simulink model "Acrobot_test"  (R2022b)
settings: Solver=FixedStepAuto  StartTime=0  StopTime=60  FixedStep=0.001  RelTol=1e-2  AbsTol=1e-3  EnableMultiTasking=on
undefined symbols (not defined in the file): AL1, AL2, Alink1_CM, Alink1_m, Alink1_MI, Alink1_PI, Alink2_CM, Alink2_m, Alink2_MI, Alink2_PI, H, W, X, Y, Z
libraries: nesl_utility x19, sm_lib x12
settings Model: Creator=李东昊  LastModifiedBy=dong
settings SolverCC: AutoScaleAbsTol=off  AlgebraicLoopSolver=TrustRegion  MaxZcPerStep=1
settings DataIOCC: LimitDataPoints=on  MaxDataPoints=10000
settings OptimizationCC: LifeSpan=inf
settings DebuggingCC: UnconnectedInputMsg=warning  UnconnectedOutputMsg=warning  UnconnectedLineMsg=warning  AllowSymbolicDim=off  SFUnexpectedBacktrackingDiag=warning  SFNoUnconditionalDefaultTransitionDiag=warning  SFExecutionAtInitializationDiag=none  SFMachineParentedDataDiag=warning  ArithmeticOperatorsInVariantConditions=warning
settings ModelReferenceCC: EnableRefExpFcnMdlSchedulingChecks=on
settings SFSimCC: SimUseLocalCustomCode=off  CustomCodeUndefinedFunction=UseInterfaceOnly
settings RTWCC: RTWUseLocalCustomCode=off  DLArmComputeVersion=19.05
settings CodeAppCC: StateflowObjectComments=on
settings GRTTargetCC: TargetLangStandard=C89/C90 (ANSI)
settings ConfigComp: CovMetricSettings=dw  CovSaveCumulativeToWorkspaceVar=on  CovSaveSingleToWorkspaceVar=on  CovExternalEMLEnable=off  CovSFcnEnable=off
settings SimscapeCC: SimscapeLogType=all  SimscapeLogSimulationStatistics=on  SimscapeLogDataHistory=10000
settings ExplorerConfigSet: InternalSimMechanicsExplorerSettings="<ExplorerConfiguration><canonicalview>aerospace</canonicalview><AnimationSetting><BasePlaybackSpeed>1.0</BasePlaybackSpeed><PlaybackSpeedFactor>1.0</PlaybackSpeedFactor></AnimationSetting><TilePanel><TileInfo><Tiles Columns=\"1\" Count=\"1\" Rows=\"1\"><Column Weight=\"1\"/><Row Weight=\"1\"/><Tile Height=\"1\" Width=\"1\" X=\"0\" Y=\"0\"/></Tiles></TileInfo><SceneInfo><SceneViewer><BGColor><R>0.60000002384185791</R><G>0.60000002384185791</G><B>0.60000002384185791</B></BGColor><Camera><DoPerspective>off</DoPerspective><Position><X>-0.471212034882517727</X><Y>0.213512906624389098</Y><Z>1.00000005247557366</Z></Position><Center><X>-0.471212034882517727</X><Y>0.213512906624389098</Y><Z>5.24755735531456935e-08</Z></Center><Up><X>0</X><Y>1</Y><Z>0</Z></Up><ViewLimDist>1</ViewLimDist><YLim>1.41406501065933288</YLim><XLim>1.62924881662923138</XLim></Camera></SceneViewer></SceneInfo></TilePanel><MechEditorPanel><Cameras/><GfxPanelCameraMap/><VideoCreator><PlaybackSpeedRatio>1.0</PlaybackSpeedRatio><FrameRate>30</FrameRate><VideoFormat>MPEG-4</VideoFormat><FrameSize>[800 600]</FrameSize></VideoCreator></MechEditorPanel></ExplorerConfiguration>"

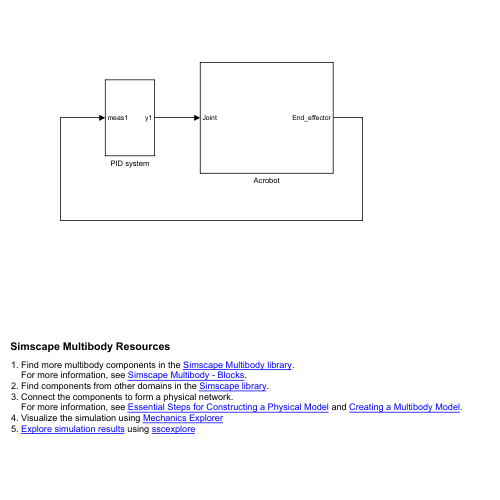
[thumbnail: Simulink's stored preview of the top-level diagram]
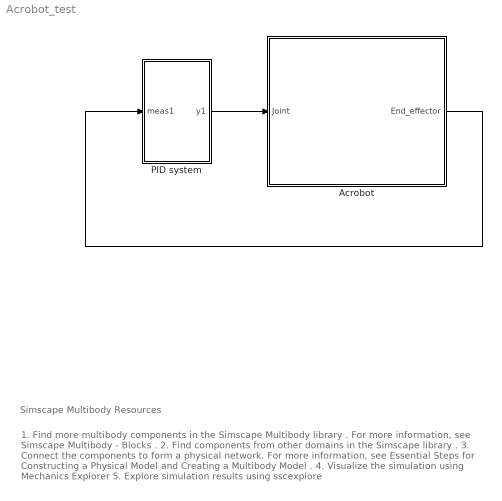
== system Acrobot_test ==
  note: 1. Find more multibody components in the Simscape Multibody library .
      | For more information, see Simscape Multibody - Blocks .
      | 2. Find components from other domains in the Simscape library .
      | 3. Connect the components to form a physical network.
      | For more information, see Essential Steps for Constructing a Physical Model and Creating a Multibody Model .
      | 4. Visualize the simulation using Mechanics Explorer
      | 5. Explore simulation results using sscexplore
  note: Simscape Multibody Resources
  Acrobot : Subsystem
  PID system : Subsystem
  wires:
  Acrobot/1(End_effector) -> PID system/1(meas1)
  PID system/1(y1) -> Acrobot/1(Joint)

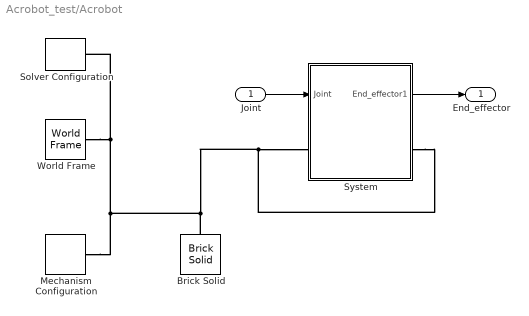
== system Acrobot_test/Acrobot ==
  Joint : Inport
  Brick Solid : sm_lib/Body Elements/Brick Solid  GraphicAmbientColor=[0.15 0.15 0.15 1.0]  BasedOnType=Density  BrickDimensions=[0.1 0.1 0.1]  BrickDimensionUnits=m  CenterOfMass=[0 0 0]  CenterOfMassUnits=m  GraphicDiffuseColor=[0.5 0.5 0.5]  Density=1000  DensityUnits=kg/m^3  DoExposeReferenceFrame=on  GraphicEmissiveColor=[0.0 0.0 0.0 1.0]  ExportEntireGeometry=off  SerializedFrames=<Frames/>  MarkerShape=Sphere  MarkerSize=10  GraphicType=FromGeometry  InertiaType=CalculateFromGeometry  Mass=1  MassUnits=kg  MomentsOfInertia=[1 1 1]  MomentsOfInertiaUnits=kg*m^2  GraphicOpacity=1.0  ProductsOfInertia=[0 0 0]  ProductsOfInertiaUnits=kg*m^2  GraphicShininess=75  GraphicSpecularColor=[0.5 0.5 0.5 1.0]  GraphicVisPropType=SimpleVisualProperties
  Mechanism Configuration : sm_lib/Utilities/Mechanism Configuration  UniformGravity=Constant  GravityVector=[0 -9.81 0]  GravityUnits=m/s^2  LinearizationDelta=0.001  JointModeTransitionNonlinearIterations=2
  Solver Configuration : nesl_utility/Solver Configuration  PhysicalDomain=network_engine_domain  SubClassName=solver  LeftPortType=input  RightPortType=generic  Tones=[]  Harmonics=[]  SimulateNoise=off  Profile=off  UseLocalSampling=off  EnableSwitchedLinearOptims=on  FrequencyDomain=off  UseCCode=off  RelTol=0.001  AbsTol=1e-06  MinStep=1e-09  ToWorkspace=off  RevertToSquareIcSolve=off  NumHomotopyIterations=100  PhasorMode=off  PhasorModeNumHarmonics=1  ConsistencySolver=NEWTON_FTOL  IndexReductionMethod=DerivativeReplacement  DoDC=off  ResidualTolerance=1e-09  ConsistencyTolSource=GLOBAL  ConsistencyAbsTol=0.001  ConsistencyRelTol=0.001  ConsistencyTolFactor=0.001  UseLocalSolver=off  LocalSolverChoice=NE_BACKWARD_EULER_ADVANCER  ResolveIndetEquations=on  FunctionEvalNumThread=1  LocalSolverSampleTime=0.001  DoFixedCost=off  MaxNonlinIter=3  MaxModeIter=2  ComputeImpulses=off  ImpulseIterations=2  LinearAlgebra=Sparse  LinearAlgebraNumThread=0  EquationFormulation=NE_TIME_EF  DelaysMemoryBudget=1024  AutomaticFiltering=on  FilteringTimeConstant=0.001  PartitionStorageMethod=AS_NEEDED  PartitionMemoryBudget=1024  PartitionMethod=FAST
  System : Subsystem
  World Frame : sm_lib/Frames and Transforms/World Frame
  End_effector : Outport
  wires:
  Joint/1 -> System/1(Joint)
  System/1(End_effector1) -> End_effector/1
  connections:
  System/LConn1 -- System/RConn1 -- Brick Solid/RConn1 -- World Frame/RConn1 -- Solver Configuration/RConn1 -- Mechanism Configuration/RConn1

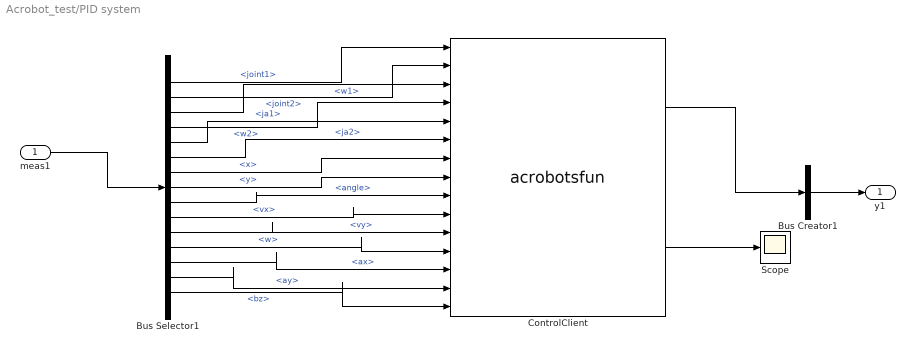
== system Acrobot_test/PID system ==
  meas1 : Inport
  Bus Creator1 : BusCreator  Inputs=1
  Bus Selector1 : BusSelector  OutputSignals=joint1,joint2,w1,w2,ja1,ja2,signal1.x,signal1.y,signal1.angle,signal1.vx,signal1.vy,signal1.w,signal1.ax,signal1.ay,signal1.bz
  ControlClient : S-Function  FunctionName=acrobotsfun  Parameters=hostname,portname,stepsize,inputnum,outputnum  SFunctionDeploymentMode=off  EnableBusSupport=off  mask{hostname=localhost, portname=8099, stepsize=0.001, inputnum=15, outputnum=2}
      mask prompts: hostname "host"; portname "port"; stepsize "step"; inputnum "input num"; outputnum "output num"
      mask DialogControl ParameterGroupVar Prompt: 参数
      mask Display:
      | color('red');
      | image('Simulink_Logo.png');
  Scope : Scope
  y1 : Outport
  wires:
  Bus Creator1/1 -> y1/1
  meas1/1 -> Bus Selector1/1
  ControlClient/1 -> Bus Creator1/1
  Bus Selector1/1 -> ControlClient/1  "<joint1>"
  Bus Selector1/2 -> ControlClient/2  "<joint2>"
  Bus Selector1/3 -> ControlClient/3  "<w1>"
  Bus Selector1/4 -> ControlClient/4  "<w2>"
  Bus Selector1/7 -> ControlClient/7  "<x>"
  Bus Selector1/8 -> ControlClient/8  "<y>"
  Bus Selector1/9 -> ControlClient/9  "<angle>"
  Bus Selector1/10 -> ControlClient/10  "<vx>"
  Bus Selector1/11 -> ControlClient/11  "<vy>"
  Bus Selector1/12 -> ControlClient/12  "<w>"
  Bus Selector1/13 -> ControlClient/13  "<ax>"
  Bus Selector1/14 -> ControlClient/14  "<ay>"
  Bus Selector1/15 -> ControlClient/15  "<bz>"
  Bus Selector1/6 -> ControlClient/6  "<ja2>"
  Bus Selector1/5 -> ControlClient/5  "<ja1>"
  ControlClient/2 -> Scope/1

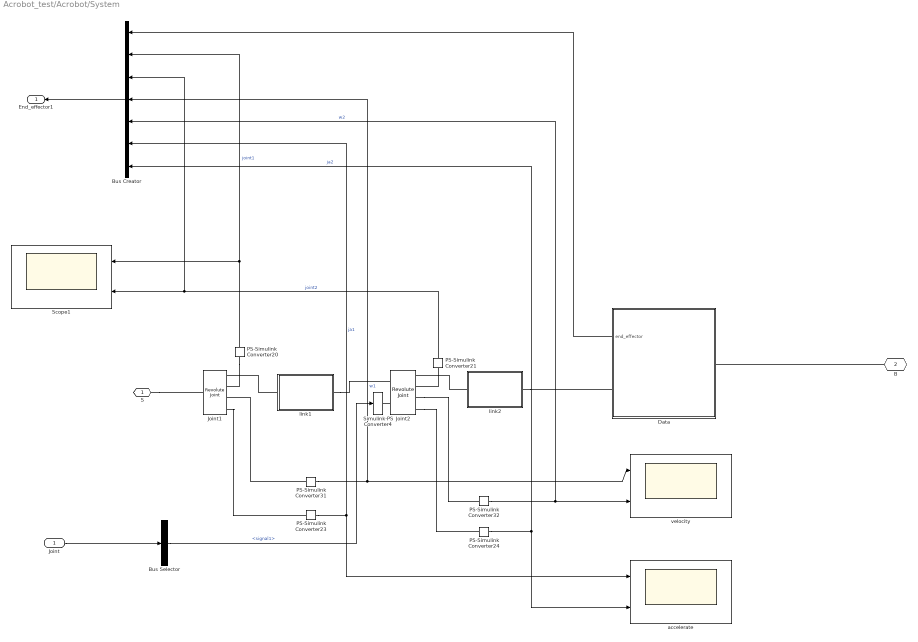
== system Acrobot_test/Acrobot/System ==
  Joint : Inport
  Bus Creator : BusCreator  Inputs=7
  Bus Selector : BusSelector  OutputSignals=signal1
  Data : Subsystem
  Joint1 : sm_lib/Joints/Revolute Joint  JointMode=Normal  SenseConstraintForce=off  SenseConstraintForceX=off  SenseConstraintForceY=off  SenseConstraintForceZ=off  SenseConstraintTorque=off  SenseConstraintTorqueX=off  SenseConstraintTorqueY=off  SenseConstraintTorqueZ=off  SenseTotalForce=off  SenseTotalForceX=off  SenseTotalForceY=off  SenseTotalForceZ=off  SenseTotalTorque=off  SenseTotalTorqueX=off  SenseTotalTorqueY=off  SenseTotalTorqueZ=off  CompositeWrenchDir=BaseOnFollower  CompositeWrenchFrame=BaseFrame  EquilibriumPosition=0  EquilibriumPositionUnits=deg  SpringStiffness=0  SpringStiffnessUnits=N*m/deg  DampingCoefficient=0  DampingCoefficientUnits=N*m/(deg/s)  TorqueActuationMode=NoTorque  MotionActuationMode=ComputedMotion  SensePosition=on  SenseVelocity=on  SenseAcceleration=on  SenseTorqueForce=off  SenseLowerLimitTorqueForce=off  SenseUpperLimitTorqueForce=off  LowerLimitSpecify=off  LowerLimitBound=-90  LowerLimitBoundUnits=deg  LowerLimitStiffness=1e4  LowerLimitStiffnessUnits=N*m/deg  LowerLimitDamping=10  LowerLimitDampingUnits=N*m/(deg/s)  LowerLimitTransitionRegionWidth=0.1  LowerLimitTransitionRegionWidthUnits=deg  UpperLimitSpecify=off  UpperLimitBound=90  UpperLimitBoundUnits=deg  UpperLimitStiffness=1e4  UpperLimitStiffnessUnits=N*m/deg  UpperLimitDamping=10  UpperLimitDampingUnits=N*m/(deg/s)  UpperLimitTransitionRegionWidth=0.1  UpperLimitTransitionRegionWidthUnits=deg  PositionTargetSpecify=off  PositionTargetPriority=High  PositionTargetValue=2.813628238  PositionTargetValueUnits=rad  VelocityTargetSpecify=off  VelocityTargetPriority=Low  VelocityTargetValue=0  VelocityTargetValueUnits=rad/s
  Joint2 : sm_lib/Joints/Revolute Joint  JointMode=Normal  SenseConstraintForce=off  SenseConstraintForceX=off  SenseConstraintForceY=off  SenseConstraintForceZ=off  SenseConstraintTorque=off  SenseConstraintTorqueX=off  SenseConstraintTorqueY=off  SenseConstraintTorqueZ=off  SenseTotalForce=off  SenseTotalForceX=off  SenseTotalForceY=off  SenseTotalForceZ=off  SenseTotalTorque=off  SenseTotalTorqueX=off  SenseTotalTorqueY=off  SenseTotalTorqueZ=off  CompositeWrenchDir=BaseOnFollower  CompositeWrenchFrame=BaseFrame  EquilibriumPosition=0  EquilibriumPositionUnits=deg  SpringStiffness=0  SpringStiffnessUnits=N*m/deg  DampingCoefficient=0  DampingCoefficientUnits=N*m/(deg/s)  TorqueActuationMode=InputTorque  MotionActuationMode=ComputedMotion  SensePosition=on  SenseVelocity=on  SenseAcceleration=on  SenseTorqueForce=off  SenseLowerLimitTorqueForce=off  SenseUpperLimitTorqueForce=off  LowerLimitSpecify=off  LowerLimitBound=-90  LowerLimitBoundUnits=rad  LowerLimitStiffness=0  LowerLimitStiffnessUnits=N*m/deg  LowerLimitDamping=0  LowerLimitDampingUnits=N*m/(deg/s)  LowerLimitTransitionRegionWidth=0.0  LowerLimitTransitionRegionWidthUnits=deg  UpperLimitSpecify=off  UpperLimitBound=90  UpperLimitBoundUnits=deg  UpperLimitStiffness=1e4  UpperLimitStiffnessUnits=N*m/deg  UpperLimitDamping=10  UpperLimitDampingUnits=N*m/(deg/s)  UpperLimitTransitionRegionWidth=0.1  UpperLimitTransitionRegionWidthUnits=deg  PositionTargetSpecify=off  PositionTargetPriority=High  PositionTargetValue=-1.48490431763342  PositionTargetValueUnits=rad  VelocityTargetSpecify=off  VelocityTargetPriority=High  VelocityTargetValue=0  VelocityTargetValueUnits=rad/s
  PS-Simulink Converter{20..21,23..24,31..32} (6 alike) : nesl_utility/PS-Simulink Converter  PhysicalDomain=network_engine_domain  SubClassName=ps_output  LeftPortType=input  RightPortType=output  PseudoPeriodic=off  Frequencies=[]  VectorFormat=inherit  Unit=inherit  AffineConversion=off
  Scope1 : Scope  NumInputPorts=2
  Simulink-PS Converter4 : nesl_utility/Simulink-PS Converter  PhysicalDomain=network_engine_domain  SubClassName=ps_input  LeftPortType=input  RightPortType=output  PseudoPeriodic=off  Frequencies=[]  NoiseDistribution=none  NoiseParameters=[]  Unit=1  AffineConversion=off  FilteringAndDerivatives=provide  SimscapeFilterOrder=2  InputFilterTimeConstant=0.001  UdotUserProvided=0
  accelerate : Scope  NumInputPorts=2
  link1 : Subsystem  mask{L=AL1, H=H, W=W, m=Alink1_m, link1_CM=Alink1_CM, link1_MI=Alink1_MI, link1_PI=Alink1_PI, rgb=[0.2 0.3 0.4]}
      mask prompts: link1_CM "Center of Mass"; link1_MI "Moments of Inertia"; link1_PI "Products of Inertia"; rgb "Color"
      mask DialogControl ParameterGroupVar Prompt: 参数
  link2 : Subsystem  mask{L=AL2, W=W, H=W, llink2_m=Alink2_m, link2_CM=Alink2_CM, link2_MI=Alink2_MI, link2_PI=Alink2_PI, rgb=[1 1 0]}
      mask prompts: llink2_m "m(kg)"; link2_CM "Center of Mass"; link2_MI "Moments of Inertia"; link2_PI "Products of Inertia"
      mask DialogControl ParameterGroupVar Prompt: 参数
  velocity : Scope  NumInputPorts=2
  S : PMIOPort  Side=Left
  B : PMIOPort  Port=2  Side=Right
  End_effector1 : Outport
  wires:
  PS-Simulink Converter23/1 -> Bus Creator/6, accelerate/1  "ja1"
  PS-Simulink Converter24/1 -> accelerate/2, Bus Creator/7  "ja2"
  PS-Simulink Converter32/1 -> Bus Creator/5, velocity/2  "w2"
  PS-Simulink Converter20/1 -> Bus Creator/2, Scope1/1  "joint1"
  PS-Simulink Converter21/1 -> Bus Creator/3, Scope1/2  "joint2"
  Bus Selector/1 -> Simulink-PS Converter4/1  "<signal1>"
  PS-Simulink Converter31/1 -> Bus Creator/4, velocity/1  "w1"
  Joint/1 -> Bus Selector/1
  Bus Creator/1 -> End_effector1/1
  Data/1(end_effector) -> Bus Creator/1
  connections:
  PS-Simulink Converter21/LConn1 -- Joint2/RConn2
  Joint2/RConn4 -- PS-Simulink Converter24/LConn1
  PS-Simulink Converter20/LConn1 -- Joint1/RConn2
  link1/LConn1 -- Joint1/RConn1
  link1/RConn1 -- Joint2/LConn1
  Joint1/RConn4 -- PS-Simulink Converter23/LConn1
  PS-Simulink Converter31/LConn1 -- Joint1/RConn3
  S/RConn1 -- Joint1/LConn1
  link2/LConn1 -- Joint2/RConn1
  Simulink-PS Converter4/RConn1 -- Joint2/LConn2
  Joint2/RConn3 -- PS-Simulink Converter32/LConn1
  B/RConn1 -- Data/LConn1
  link2/RConn1 -- Data/RConn1

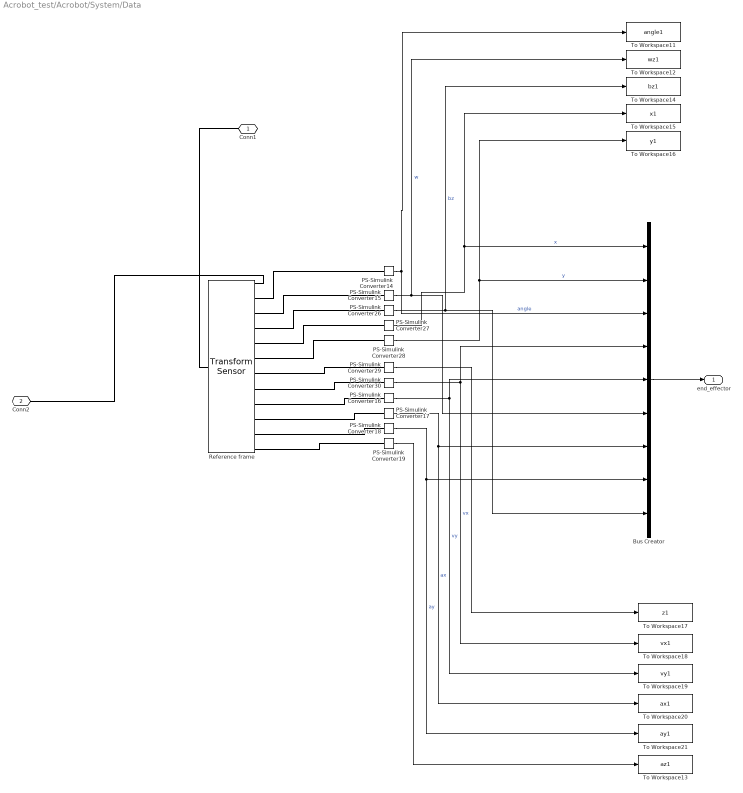
== system Acrobot_test/Acrobot/System/Data ==
  Bus Creator : BusCreator  Inputs=9
  PS-Simulink Converter{14..19,26..30} (11 alike) : nesl_utility/PS-Simulink Converter  PhysicalDomain=network_engine_domain  SubClassName=ps_output  LeftPortType=input  RightPortType=output  PseudoPeriodic=off  Frequencies=[]  VectorFormat=inherit  Unit=inherit  AffineConversion=off
  Reference frame : sm_lib/Frames and Transforms/Transform Sensor  MeasurementFrame=Base  SenseAngle=on  SenseAxis=off  SenseQ=off  SenseR=off  SenseRotationSequence=off  RotationSequence=XYX  SenseOmegaX=off  SenseOmegaY=off  SenseOmegaZ=on  SenseQDot=off  SenseRDot=off  SenseAlphaX=off  SenseAlphaY=off  SenseAlphaZ=on  SenseQDDot=off  SenseRDDot=off  SenseX=on  SenseY=on  SenseZ=on  SenseRad=off  SenseAzim=off  SenseDist=off  SenseInc=off  SenseXDot=on  SenseYDot=on  SenseZDot=off  SenseRadDot=off  SenseAzimDot=off  SenseDistDot=off  SenseIncDot=off  SenseXDDot=on  SenseYDDot=on  SenseZDDot=on  SenseRadDDot=off  SenseAzimDDot=off  SenseDistDDot=off  SenseIncDDot=off
  To Workspace11 : ToWorkspace  VariableName=angle1  SaveFormat=Structure With Time  SampleTime=-1
  To Workspace12 : ToWorkspace  VariableName=wz1  SaveFormat=Structure With Time  SampleTime=-1
  To Workspace13 : ToWorkspace  VariableName=az1  SaveFormat=Structure With Time  SampleTime=-1
  To Workspace14 : ToWorkspace  VariableName=bz1  SaveFormat=Structure With Time  SampleTime=-1
  To Workspace15 : ToWorkspace  VariableName=x1  SaveFormat=Structure With Time  SampleTime=-1
  To Workspace16 : ToWorkspace  VariableName=y1  SaveFormat=Structure With Time  SampleTime=-1
  To Workspace17 : ToWorkspace  VariableName=z1  SaveFormat=Structure With Time  SampleTime=-1
  To Workspace18 : ToWorkspace  VariableName=vx1  SaveFormat=Structure With Time  SampleTime=-1
  To Workspace19 : ToWorkspace  VariableName=vy1  SaveFormat=Structure With Time  SampleTime=-1
  To Workspace20 : ToWorkspace  VariableName=ax1  SaveFormat=Structure With Time  SampleTime=-1
  To Workspace21 : ToWorkspace  VariableName=ay1  SaveFormat=Structure With Time  SampleTime=-1
  Conn1 : PMIOPort  Side=Left
  Conn2 : PMIOPort  Port=2  Side=Right
  end_effector : Outport
  wires:
  PS-Simulink Converter26/1 -> Bus Creator/9, To Workspace14/1  "bz"
  PS-Simulink Converter17/1 -> Bus Creator/7, To Workspace20/1  "ax"
  PS-Simulink Converter18/1 -> Bus Creator/8, To Workspace21/1  "ay"
  PS-Simulink Converter15/1 -> Bus Creator/6, To Workspace12/1  "w"
  PS-Simulink Converter27/1 -> Bus Creator/1, To Workspace15/1  "x"
  PS-Simulink Converter29/1 -> To Workspace17/1
  PS-Simulink Converter19/1 -> To Workspace13/1
  PS-Simulink Converter14/1 -> To Workspace11/1, Bus Creator/3  "angle"
  PS-Simulink Converter16/1 -> Bus Creator/5, To Workspace19/1  "vy"
  PS-Simulink Converter28/1 -> Bus Creator/2, To Workspace16/1  "y"
  PS-Simulink Converter30/1 -> Bus Creator/4, To Workspace18/1  "vx"
  Bus Creator/1 -> end_effector/1
  connections:
  Reference frame/RConn3 -- PS-Simulink Converter15/LConn1
  Reference frame/RConn7 -- PS-Simulink Converter29/LConn1
  Reference frame/RConn6 -- PS-Simulink Converter28/LConn1
  Reference frame/RConn8 -- PS-Simulink Converter30/LConn1
  Reference frame/RConn9 -- PS-Simulink Converter16/LConn1
  Reference frame/RConn11 -- PS-Simulink Converter18/LConn1
  Reference frame/RConn4 -- PS-Simulink Converter26/LConn1
  PS-Simulink Converter14/LConn1 -- Reference frame/RConn2
  Reference frame/RConn10 -- PS-Simulink Converter17/LConn1
  Reference frame/RConn5 -- PS-Simulink Converter27/LConn1
  Reference frame/RConn1 -- Conn2/RConn1
  Conn1/RConn1 -- Reference frame/LConn1
  Reference frame/RConn12 -- PS-Simulink Converter19/LConn1

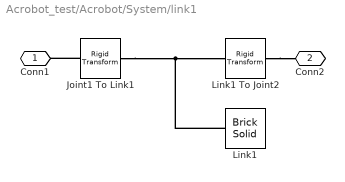
== system Acrobot_test/Acrobot/System/link1 ==
  Joint1 To Link1 : sm_lib/Frames and Transforms/Rigid Transform  TranslationMethod=None  TranslationStandardOffset=L/2  TranslationLengthUnit=m  TranslationStandardAxis=+Y  TranslationCartesianOffset=[0 0 0]  TranslationROffset=0  TranslationROffsetUnits=m  TranslationZOffset=0  TranslationZOffsetUnits=m  TranslationThetaOffset=0  TranslationThetaOffsetUnits=deg  RotationMethod=StandardAxis  RotationAngleUnits=deg  RotationStandardAxis=+Z  RotationAngle=90  RotationArbitraryAxis=[0 0 1]  FollAlignAxisA=+X  BaseAlignAxisA=+Y  FollAlignAxisB=+Y  BaseAlignAxisB=+Z  RotationSequenceAxes=FollowerAxes  RotationSequence=XYX  RotationSequenceAngles=[0 0 0]  RotationSequenceAnglesUnits=deg  RotationMatrix=[1 0 0; 0 1 0; 0 0 1]  Quaternion=[1 0 0 0]
  Link1 : sm_lib/Body Elements/Brick Solid  GraphicAmbientColor=[0.15 0.15 0.15 1.0]  BasedOnType=Density  BrickDimensions=[L H W]  BrickDimensionUnits=m  CenterOfMass=Alink1_CM  CenterOfMassUnits=m  GraphicDiffuseColor=rgb  Density=rho  DensityUnits=kg/m^3  DoExposeReferenceFrame=off  GraphicEmissiveColor=[0.0 0.0 0.0 1.0]  ExportEntireGeometry=off  SerializedFrames=<Frames><Frame><Id>Frame1</Id><Value><Name>F1</Name><Origin><Source>GeometricFeature</Source><FeatureName>-x surface</FeatureName></Origin><PrimaryAxis><DefinedDirection>+Y</DefinedDirection><Source>ReferenceFrame</Source><SourceDirection>+Y</SourceDirection><FeatureName></FeatureName></PrimaryAxis><SecondaryAxis><DefinedDirection>+X</DefinedDirection><Source>ReferenceFrame</Source><SourceDirection>+X</SourceDirection><FeatureName></FeatureName></SecondaryAxis></Value></Frame></Frames>  MarkerShape=Sphere  MarkerSize=10  GraphicType=FromGeometry  InertiaType=Custom  Mass=Alink1_m  MassUnits=kg  MomentsOfInertia=Alink1_MI  MomentsOfInertiaUnits=kg*m^2  GraphicOpacity=1.0  ProductsOfInertia=Alink1_PI  ProductsOfInertiaUnits=kg*m^2  GraphicShininess=75  GraphicSpecularColor=[0.5 0.5 0.5 1.0]  GraphicVisPropType=SimpleVisualProperties
  Link1 To Joint2 : sm_lib/Frames and Transforms/Rigid Transform  TranslationMethod=StandardAxis  TranslationStandardOffset=AL1  TranslationLengthUnit=m  TranslationStandardAxis=+X  TranslationCartesianOffset=[0 0 0]  TranslationROffset=0  TranslationROffsetUnits=m  TranslationZOffset=0  TranslationZOffsetUnits=m  TranslationThetaOffset=0  TranslationThetaOffsetUnits=deg  RotationMethod=None  RotationAngleUnits=deg  RotationStandardAxis=+Z  RotationAngle=0.0  RotationArbitraryAxis=[0 0 1]  FollAlignAxisA=+X  BaseAlignAxisA=+Y  FollAlignAxisB=+Y  BaseAlignAxisB=+Z  RotationSequenceAxes=FollowerAxes  RotationSequence=XYX  RotationSequenceAngles=[0 0 0]  RotationSequenceAnglesUnits=deg  RotationMatrix=[1 0 0; 0 1 0; 0 0 1]  Quaternion=[1 0 0 0]
  Conn1 : PMIOPort  Side=Left
  Conn2 : PMIOPort  Port=2  Side=Right
  connections:
  Joint1 To Link1/RConn1 -- Link1/LConn1 -- Link1 To Joint2/LConn1
  Joint1 To Link1/LConn1 -- Conn1/RConn1
  Link1 To Joint2/RConn1 -- Conn2/RConn1

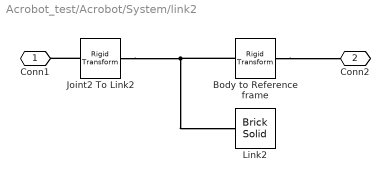
== system Acrobot_test/Acrobot/System/link2 ==
  Body to Reference frame : sm_lib/Frames and Transforms/Rigid Transform  TranslationMethod=StandardAxis  TranslationStandardOffset=AL2  TranslationLengthUnit=m  TranslationStandardAxis=+X  TranslationCartesianOffset=[0 0 0]  TranslationROffset=0  TranslationROffsetUnits=m  TranslationZOffset=0  TranslationZOffsetUnits=m  TranslationThetaOffset=0  TranslationThetaOffsetUnits=deg  RotationMethod=None  RotationAngleUnits=deg  RotationStandardAxis=-Z  RotationAngle=90  RotationArbitraryAxis=[0 0 1]  FollAlignAxisA=+X  BaseAlignAxisA=+Y  FollAlignAxisB=+Y  BaseAlignAxisB=+Z  RotationSequenceAxes=FollowerAxes  RotationSequence=XYX  RotationSequenceAngles=[0 0 0]  RotationSequenceAnglesUnits=deg  RotationMatrix=[1 0 0; 0 1 0; 0 0 1]  Quaternion=[1 0 0 0]
  Joint2 To Link2 : sm_lib/Frames and Transforms/Rigid Transform  TranslationMethod=None  TranslationStandardOffset=L/2  TranslationLengthUnit=m  TranslationStandardAxis=+X  TranslationCartesianOffset=[0 0 0]  TranslationROffset=0  TranslationROffsetUnits=m  TranslationZOffset=0  TranslationZOffsetUnits=m  TranslationThetaOffset=0  TranslationThetaOffsetUnits=deg  RotationMethod=None  RotationAngleUnits=deg  RotationStandardAxis=+Z  RotationAngle=0.0  RotationArbitraryAxis=[0 0 1]  FollAlignAxisA=+X  BaseAlignAxisA=+Y  FollAlignAxisB=+Y  BaseAlignAxisB=+Z  RotationSequenceAxes=FollowerAxes  RotationSequence=XYX  RotationSequenceAngles=[0 0 0]  RotationSequenceAnglesUnits=deg  RotationMatrix=[1 0 0; 0 1 0; 0 0 1]  Quaternion=[1 0 0 0]
  Link2 : sm_lib/Body Elements/Brick Solid  GraphicAmbientColor=[0.15 0.15 0.15 1.0]  BasedOnType=Density  BrickDimensions=[L H W]  BrickDimensionUnits=m  CenterOfMass=Alink2_CM  CenterOfMassUnits=m  GraphicDiffuseColor=rgb  Density=rho  DensityUnits=kg/m^3  DoExposeReferenceFrame=off  GraphicEmissiveColor=[0.0 0.0 0.0 1.0]  ExportEntireGeometry=off  SerializedFrames=<Frames><Frame><Id>Frame1</Id><Value><Name>F1</Name><Origin><Source>GeometricFeature</Source><FeatureName>-x surface</FeatureName></Origin><PrimaryAxis><DefinedDirection>+Z</DefinedDirection><Source>ReferenceFrame</Source><SourceDirection>+Z</SourceDirection><FeatureName></FeatureName></PrimaryAxis><SecondaryAxis><DefinedDirection>+X</DefinedDirection><Source>ReferenceFrame</Source><SourceDirection>+X</SourceDirection><FeatureName></FeatureName></SecondaryAxis></Value></Frame></Frames>  MarkerShape=Sphere  MarkerSize=10  GraphicType=FromGeometry  InertiaType=Custom  Mass=Alink2_m  MassUnits=kg  MomentsOfInertia=Alink2_MI  MomentsOfInertiaUnits=kg*m^2  GraphicOpacity=1.0  ProductsOfInertia=Alink2_PI  ProductsOfInertiaUnits=kg*m^2  GraphicShininess=75  GraphicSpecularColor=[0.5 0.5 0.5 1.0]  GraphicVisPropType=SimpleVisualProperties
  Conn1 : PMIOPort  Side=Left
  Conn2 : PMIOPort  Port=2  Side=Right
  connections:
  Joint2 To Link2/RConn1 -- Body to Reference frame/LConn1 -- Link2/LConn1
  Joint2 To Link2/LConn1 -- Conn1/RConn1
  Body to Reference frame/RConn1 -- Conn2/RConn1
